simulink model "BMO_sfun"  (R2015b)
settings: Solver=FixedStepDiscrete  StartTime=0.0  StopTime=inf  RelTol=1e-3
undefined symbols (not defined in the file): BMOk_BatteryCurrentThresh
settings Model: TunableVars=BMOk_BatteryCurrentThresh,BMOk_CcClosing,BMOk_CcOpening,BMOk_Charging,BMOk_ChargingSleep,BMOk_Discharging,BMOk_Off,BMOk_On,BMOk_PowerClosed,BMOk_PowerOff,BMOk_PowerOn  TunableVarsStorageClass=Auto,Auto,Auto,Auto,Auto,Auto,Auto,Auto,Auto,Auto,Auto  TunableVarsTypeQualifier=,,,,,,,,,,  Creator=nctzv8  LastModifiedBy=nctzv8
settings ConfigSet: Description=OpenECU configuration set for code generation under RTW-EC.
settings SolverCC: PositivePriorityOrder=on
settings DataIOCC: SaveFormat=Array  SignalLoggingSaveFormat=ModelDataLogs
settings OptimizationCC: DefaultParameterBehavior=Inlined  InlineInvariantSignals=on  ExpressionDepthLimit=2147483647  StateBitsets=on  DataBitsets=on  ZeroExternalMemoryAtStartup=off  ZeroInternalMemoryAtStartup=off  NoFixptDivByZeroProtection=on  EfficientFloat2IntCast=on  OptimizeModelRefInitCode=on  LifeSpan=1
settings DebuggingCC: SaveWithParameterizedLinksMsg=none  UnderspecifiedInitializationDetection=Classic  MergeDetectMultiDrivingBlocksExec=none  SignalResolutionControl=TryResolveAllWithWarning  MultiTaskDSMMsg=warning  MultiTaskCondExecSysMsg=none  SingleTaskRateTransMsg=error  CheckMatrixSingularityMsg=warning  VectorMatrixConversionMsg=warning  FcnCallInpInsideContextMsg=UseLocalSettings  SignalLabelMismatchMsg=warning  StateNameClashWarn=warning  StrictBusMsg=None
settings HardwareCC: ProdBitPerPointer=32  ProdLargestAtomicInteger=Long  ProdLargestAtomicFloat=Double  ProdEndianess=BigEndian  ProdWordSize=32  ProdHWDeviceType=Freescale->32-bit PowerPC  TargetIntDivRoundTo=Zero  TargetEndianess=BigEndian  TargetHWDeviceType=Freescale->32-bit PowerPC  ProdEqTarget=off
settings RTWCC: SystemTargetFile=openecu_ert.tlc  MakeCommand=make_rtw optimized_floating_point=1  TemplateMakefile=openecu_ert_r2015b_64.tmf  Description=OpenECU Platform Target (ERT, optimised floating-point code)  RetainRTWFile=on  IncludeHyperlinkInReport=on
settings CodeAppCC: ForceParamTrailComments=on  IgnoreCustomStorageClasses=off  SimulinkDataObjDesc=on  CustomSymbolStrType=$N$R$M  InsertBlockDesc=on  InternalIdentifier=Classic
settings STFCustomTargetCC: TargetLibSuffix=.a  GenerateSampleERTMain=on  ConcurrentExecutionCompliant=off  IncludeMdlTerminateFcn=off  GeneratePreprocessorConditionals=Use local settings  CombineOutputUpdateFcns=on  IncludeFileDelimiter=UseQuote  ERTCustomFileBanners=on  SupportContinuousTime=off  MATLABClassNameForMDSCustomization=Simulink.SoftwareTarget.ERTCustomization  CPPClassGenCompliant=off  GRTInterface=off  SystemTargetFile=openecu_ert.tlc
settings ERTTargetCC: GenerateSampleERTMain=on  ParMdlRefBuildCompliant=off  CompOptLevelCompliant=off  ConcurrentExecutionCompliant=off  IncludeMdlTerminateFcn=off  ERTFirstTimeCompliant=off  IncludeFileDelimiter=UseQuote  SupportNonInlinedSFcns=on  ModelStepFunctionPrototypeControlCompliant=off  CPPClassGenCompliant=off  UseToolchainInfoCompliant=off  ExtModeMexFile=noextcomm  InlinedParameterPlacement=NonHierarchical  ERTSrcFileBannerTemplate=oe_code_c_template.cgt  ERTHdrFileBannerTemplate=oe_code_h_template.cgt  ERTDataSrcFileTemplate=oe_data_c_template.cgt  ERTDataHdrFileTemplate=oe_data_h_template.cgt  ERTCustomFileTemplate=example_file_process.tlc  GlobalDataDefinition=InSeparateSourceFile  GlobalDataReference=InSeparateHeaderFile  EnableUserReplacementTypes=on

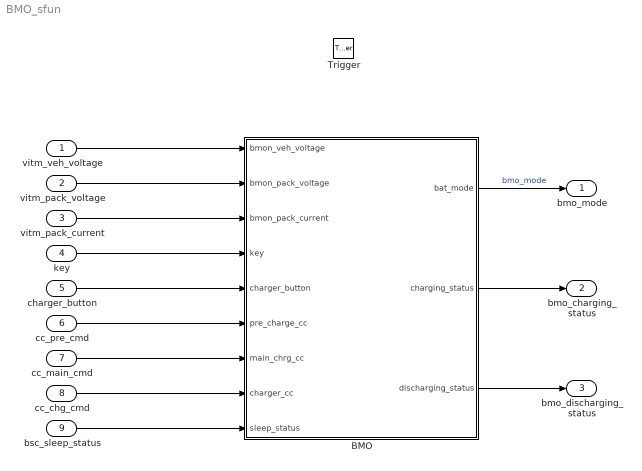
== system BMO_sfun ==
  vitm_veh_voltage : Inport
  vitm_pack_voltage : Inport  Port=2
  vitm_pack_current : Inport  Port=3
  key : Inport  Port=4  OutDataTypeStr=uint8
  charger_button : Inport  Port=5  OutDataTypeStr=uint8
  cc_pre_cmd : Inport  Port=6
  cc_main_cmd : Inport  Port=7
  cc_chg_cmd : Inport  Port=8  OutDataTypeStr=boolean
  bsc_sleep_status : Inport  Port=9  OutDataTypeStr=boolean
  Trigger : TriggerPort  TriggerType=function-call  PortDimensions=1
  BMO : Subsystem  mask{sfcnParam1=BMOk_BatteryCurrentThresh}
      mask prompts: sfcnParam1 "BMOk_BatteryCurrentThresh:"
      mask help: Simulink:masks:GenSFuncDesc_MD
      mask Help: eval('feval(''rtwprivate'',''rtwhelpview'',''rtw_sfcn_block'')');
  bmo_mode : Outport
  bmo_charging_status : Outport  Port=2
  bmo_discharging_status : Outport  Port=3
  wires:
  vitm_veh_voltage/1 -> BMO/1(bmon_veh_voltage)
  vitm_pack_voltage/1 -> BMO/2(bmon_pack_voltage)
  vitm_pack_current/1 -> BMO/3(bmon_pack_current)
  key/1 -> BMO/4(key)
  cc_pre_cmd/1 -> BMO/6(pre_charge_cc)
  bsc_sleep_status/1 -> BMO/9(sleep_status)
  cc_chg_cmd/1 -> BMO/8(charger_cc)
  cc_main_cmd/1 -> BMO/7(main_chrg_cc)
  charger_button/1 -> BMO/5(charger_button)
  BMO/1(bat_mode) -> bmo_mode/1  "bmo_mode"
  BMO/2(charging_status) -> bmo_charging_status/1
  BMO/3(discharging_status) -> bmo_discharging_status/1

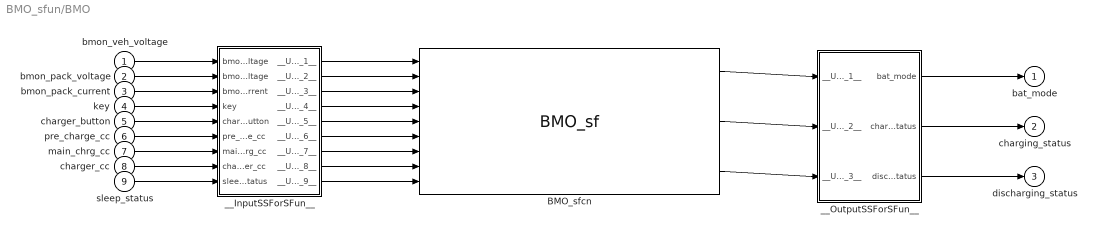
== system BMO_sfun/BMO ==
  bmon_veh_voltage : Inport
  bmon_pack_voltage : Inport  Port=2
  bmon_pack_current : Inport  Port=3
  key : Inport  Port=4
  charger_button : Inport  Port=5
  pre_charge_cc : Inport  Port=6
  main_chrg_cc : Inport  Port=7
  charger_cc : Inport  Port=8
  sleep_status : Inport  Port=9
  BMO_sfcn : S-Function  FunctionName=BMO_sf  Parameters=sfcnParam1  SFunctionModules=""  SFunctionDeploymentMode=off  EnableBusSupport=off  mask{rtw_sf_name=BMO_sf, showVar=off, sfcnParam1=sfcnParam1}
      mask prompts: rtw_sf_name "Simulink:masks:GenSFuncName_MP"; showVar "Simulink:masks:GenSFuncShowModuleList_MP"; sfcnParam1 "BMOk_BatteryCurrentThresh:"
      mask help: Simulink:masks:GenSFuncDesc_MD
      mask init:
      | displist = '';
      | if ~strcmp(get_param(gcb, 'FunctionName'), rtw_sf_name);
      |   set_param(gcb, 'FunctionName', rtw_sf_name);
      | end
      | % Check if we are generating code
      | rtw_mode = false;
      | if strcmpi(get_param(bdroot(gcb),'SimulationStatus'),'Initializing')
      | 	rtw_mode = strcmpi(get_param(bdroot(gcb),'BuildingRTWCode'),'on') && ...
      | 		~strcmpi(get_param(bdroot(gcb),'TargetStyle'),'SimulationTarget');
      | end
      | if showVar || rtw_mode
      | 	if exist('rtwsfunc') == 2 | exist('rtwsfunc') == 6
      | 		tmplist = rtwsfunc(rtw_sf_name,gcb);
      | 		tmplist = DAStudio.message('Simulink:masks:GenSFuncListOfModules_IC', tmplist);
      | 	elseif showVar
      | 		tmplist1 = DAStudio.message('Simulink:masks:GenSFuncListOfModules_IC', '');
      |         tmplist2 = DAStudio.message('Simulink:masks:GenSFuncNotLicensed_IC');
      |         tmplist = [tmplist1 tmplist2];
      |  	end
      | end
      | if showVar
      |   displist = tmplist;
      | end
      settings: CopyFcn=|
      | if ~strcmp(get_param(gcb,'Linkstatus'),'none') && ...
      | ~strcmp(get_param(gcb,'Linkstatus'),'implicit')
      |   set_param(gcb,'LinkStatus','none');
      | end
      mask Help: eval('feval(''rtwprivate'',''rtwhelpview'',''rtw_sfcn_block'')');
      mask Display:
      | port_label('input',1,'bmon_veh_voltage');
      | port_label('input',2,'bmon_pack_voltage');
      | port_label('input',3,'bmon_pack_current');
      | port_label('input',4,'key');
      | port_label('input',5,'charger_button');
      | port_label('input',6,'pre_charge_cc');
      | port_label('input',7,'main_chrg_cc');
      | port_label('input',8,'charger_cc');
      | port_label('input',9,'sleep_status');
      | port_label('output',1,'bat_mode');
      | port_label('output',2,'charging_status');
      | port_label('output',3,'discharging_status');
  __InputSSForSFun__ : Subsystem
  __OutputSSForSFun__ : Subsystem
  bat_mode : Outport
  charging_status : Outport  Port=2
  discharging_status : Outport  Port=3
  wires:
  bmon_veh_voltage/1 -> __InputSSForSFun__/1(bmon_veh_voltage)
  bmon_pack_voltage/1 -> __InputSSForSFun__/2(bmon_pack_voltage)
  bmon_pack_current/1 -> __InputSSForSFun__/3(bmon_pack_current)
  key/1 -> __InputSSForSFun__/4(key)
  charger_button/1 -> __InputSSForSFun__/5(charger_button)
  pre_charge_cc/1 -> __InputSSForSFun__/6(pre_charge_cc)
  main_chrg_cc/1 -> __InputSSForSFun__/7(main_chrg_cc)
  charger_cc/1 -> __InputSSForSFun__/8(charger_cc)
  sleep_status/1 -> __InputSSForSFun__/9(sleep_status)
  __InputSSForSFun__/1(__UniqueOutportName__1__) -> BMO_sfcn/1
  __InputSSForSFun__/2(__UniqueOutportName__2__) -> BMO_sfcn/2
  __InputSSForSFun__/3(__UniqueOutportName__3__) -> BMO_sfcn/3
  __InputSSForSFun__/4(__UniqueOutportName__4__) -> BMO_sfcn/4
  __InputSSForSFun__/5(__UniqueOutportName__5__) -> BMO_sfcn/5
  __InputSSForSFun__/6(__UniqueOutportName__6__) -> BMO_sfcn/6
  __InputSSForSFun__/7(__UniqueOutportName__7__) -> BMO_sfcn/7
  __InputSSForSFun__/8(__UniqueOutportName__8__) -> BMO_sfcn/8
  __InputSSForSFun__/9(__UniqueOutportName__9__) -> BMO_sfcn/9
  BMO_sfcn/1 -> __OutputSSForSFun__/1(__UniqueInportName__1__)
  BMO_sfcn/2 -> __OutputSSForSFun__/2(__UniqueInportName__2__)
  BMO_sfcn/3 -> __OutputSSForSFun__/3(__UniqueInportName__3__)
  __OutputSSForSFun__/1(bat_mode) -> bat_mode/1
  __OutputSSForSFun__/2(charging_status) -> charging_status/1
  __OutputSSForSFun__/3(discharging_status) -> discharging_status/1

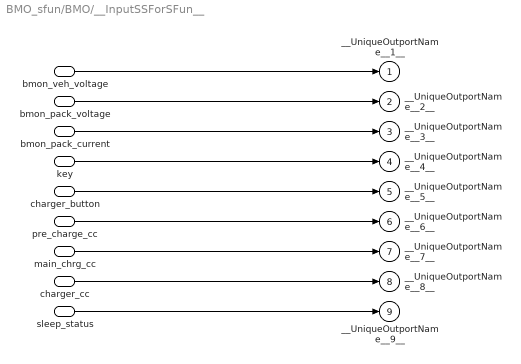
== system BMO_sfun/BMO/__InputSSForSFun__ ==
  bmon_veh_voltage : Inport
  bmon_pack_voltage : Inport  Port=2
  bmon_pack_current : Inport  Port=3
  key : Inport  Port=4
  charger_button : Inport  Port=5
  pre_charge_cc : Inport  Port=6
  main_chrg_cc : Inport  Port=7
  charger_cc : Inport  Port=8
  sleep_status : Inport  Port=9
  __UniqueOutportName__1__ : Outport
  __UniqueOutportName__2__ : Outport  Port=2
  __UniqueOutportName__3__ : Outport  Port=3
  __UniqueOutportName__4__ : Outport  Port=4
  __UniqueOutportName__5__ : Outport  Port=5
  __UniqueOutportName__6__ : Outport  Port=6
  __UniqueOutportName__7__ : Outport  Port=7
  __UniqueOutportName__8__ : Outport  Port=8
  __UniqueOutportName__9__ : Outport  Port=9
  wires:
  bmon_veh_voltage/1 -> __UniqueOutportName__1__/1
  bmon_pack_voltage/1 -> __UniqueOutportName__2__/1
  bmon_pack_current/1 -> __UniqueOutportName__3__/1
  key/1 -> __UniqueOutportName__4__/1
  charger_button/1 -> __UniqueOutportName__5__/1
  pre_charge_cc/1 -> __UniqueOutportName__6__/1
  main_chrg_cc/1 -> __UniqueOutportName__7__/1
  charger_cc/1 -> __UniqueOutportName__8__/1
  sleep_status/1 -> __UniqueOutportName__9__/1

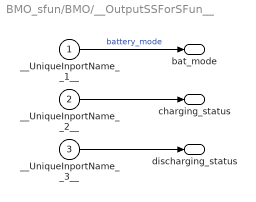
== system BMO_sfun/BMO/__OutputSSForSFun__ ==
  __UniqueInportName__1__ : Inport
  __UniqueInportName__2__ : Inport  Port=2
  __UniqueInportName__3__ : Inport  Port=3
  bat_mode : Outport
  charging_status : Outport  Port=2
  discharging_status : Outport  Port=3
  wires:
  __UniqueInportName__1__/1 -> bat_mode/1  "battery_mode"
  __UniqueInportName__2__/1 -> charging_status/1
  __UniqueInportName__3__/1 -> discharging_status/1
